simulink model "DC_motor_model"  (R2025b)
settings: Solver=VariableStepAuto  StartTime=0.0  StopTime=10.0  RelTol=1e-3
undefined symbols (not defined in the file or in its folder): b, J, K, L, R
settings Model: Creator=REARDONNM24  LastModifiedBy=REARDONNM24

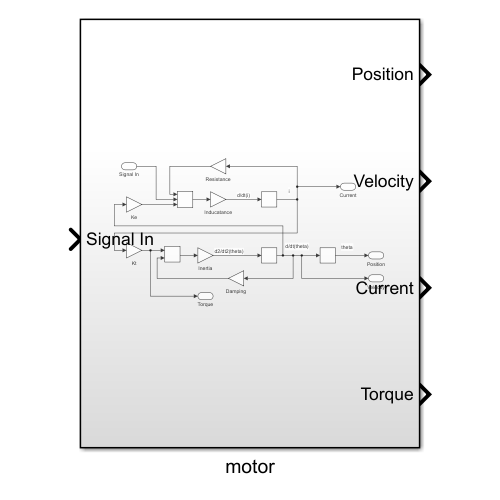
[thumbnail: Simulink's stored preview of the top-level diagram]
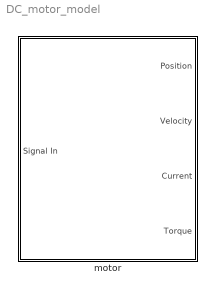
== system DC_motor_model ==
  motor : Subsystem

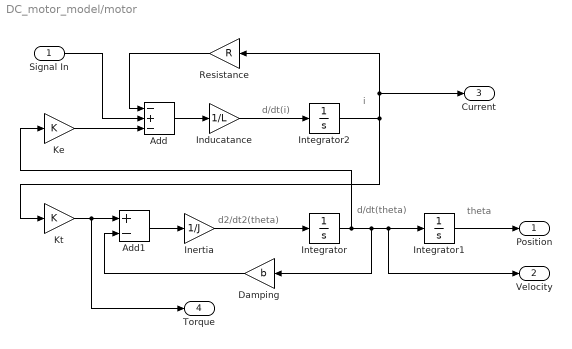
== system DC_motor_model/motor ==
  note: i
  note: d/dt(i)
  note: theta
  note: d/dt(theta)
  note: d2/dt2(theta)
  Signal In : Inport
  Add : Sum  Inputs=-+-
  Add1 : Sum  Inputs=+-
  Damping : Gain  Gain=b
  Inducatance : Gain  Gain=1/L
  Inertia : Gain  Gain=1/J
  Integrator : Integrator
  Integrator1 : Integrator
  Integrator2 : Integrator
  Ke : Gain  Gain=K
  Kt : Gain  Gain=K
  Resistance : Gain  Gain=R
  Position : Outport
  Velocity : Outport  Port=2
  Current : Outport  Port=3
  Torque : Outport  Port=4
  wires:
  Signal In/1 -> Add/2
  Resistance/1 -> Add/1
  Inertia/1 -> Integrator/1
  Integrator/1 -> Ke/1, Damping/1, Velocity/1, Integrator1/1
  Integrator2/1 -> Kt/1, Current/1, Resistance/1
  Damping/1 -> Add1/2
  Inducatance/1 -> Integrator2/1
  Add1/1 -> Inertia/1
  Add/1 -> Inducatance/1
  Kt/1 -> Torque/1, Add1/1
  Ke/1 -> Add/3
  Integrator1/1 -> Position/1
